simulink model "strelkowa_rep3_ODE"  (R2013a)
settings: Solver=ode4  StartTime=0.0  StopTime=3000.0  FixedStep=0.1  RelTol=1e-3
values from neighbouring files (symbols this model uses):
  c1 = P1(a)    [evaluation_ODE.m]    (also in init_Strelkowa_ODE.m = 1.6)
  c2 = 0.12    [evaluation_ODE.m]    (also in init_Strelkowa_ODE.m)
  c3 = 2.6    [evaluation_ODE.m]    (also in init_Strelkowa_ODE.m)
  c4 = 0.06    [evaluation_ODE.m]    (also in init_Strelkowa_ODE.m)
  mRNA_init = 10    [evaluation_ODE.m]    (also in init_Strelkowa_ODE.m)
settings Model: Creator=Jure Bordon  LastModifiedBy=Jure Bordon

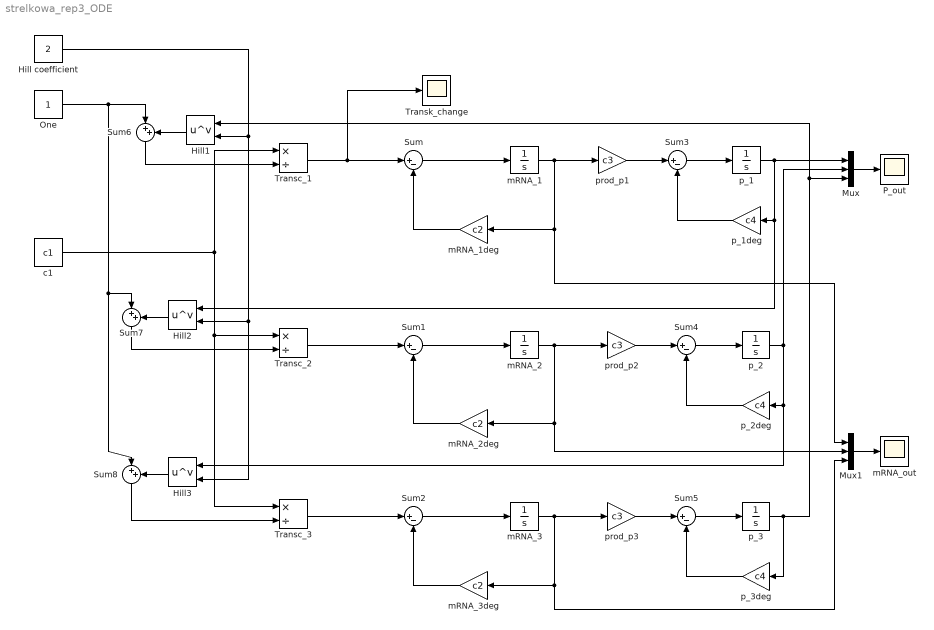
== system strelkowa_rep3_ODE ==
  Hill coefficient : Constant  Value=2
  Hill1 : Math  Operator=pow  SaturateOnIntegerOverflow=on
  Hill2 : Math  Operator=pow  SaturateOnIntegerOverflow=on
  Hill3 : Math  Operator=pow  SaturateOnIntegerOverflow=on
  Mux : Mux  Inputs=3
  Mux1 : Mux  Inputs=3
  One : Constant
  P_out : Scope
      settings: SaveName=P_out_ODE
  Sum{,1..5} (6 alike) : Sum  Inputs=|+-
  Sum6 : Sum  Inputs=|++
  Sum7 : Sum  Inputs=|++
  Sum8 : Sum  Inputs=|++
  Transc_1 : Product  Inputs=*/
  Transc_2 : Product  Inputs=*/
  Transc_3 : Product  Inputs=*/
  Transk_change : Scope
      settings: SaveName=P_out
  c1 : Constant  Value=c1
  mRNA_1 : Integrator  InitialCondition=mRNA_init + 0.5
  mRNA_1deg : Gain  Gain=c2
  mRNA_2 : Integrator  InitialCondition=mRNA_init
  mRNA_2deg : Gain  Gain=c2
  mRNA_3 : Integrator  InitialCondition=mRNA_init
  mRNA_3deg : Gain  Gain=c2
  mRNA_out : Scope
      settings: SaveName=mRNA_out_ODE
  p_1 : Integrator
  p_1deg : Gain  Gain=c4
  p_2 : Integrator
  p_2deg : Gain  Gain=c4
  p_3 : Integrator
  p_3deg : Gain  Gain=c4
  prod_p1 : Gain  Gain=c3
  prod_p2 : Gain  Gain=c3
  prod_p3 : Gain  Gain=c3
  wires:
  Sum/1 -> mRNA_1/1
  Sum1/1 -> mRNA_2/1
  Sum2/1 -> mRNA_3/1
  Sum3/1 -> p_1/1
  p_1/1 -> Mux/1, Hill2/1, p_1deg/1
  p_1deg/1 -> Sum3/2
  Sum4/1 -> p_2/1
  p_2/1 -> p_2deg/1, Hill3/1, Mux/2
  p_2deg/1 -> Sum4/2
  Sum5/1 -> p_3/1
  p_3/1 -> p_3deg/1, Hill1/1, Mux/3
  p_3deg/1 -> Sum5/2
  Sum6/1 -> Transc_1/2
  Sum8/1 -> Transc_3/2
  One/1 -> Sum7/1, Sum8/1, Sum6/1
  Transc_3/1 -> Sum2/1
  Transc_2/1 -> Sum1/1
  Transc_1/1 -> Transk_change/1, Sum/1
  Sum7/1 -> Transc_2/2
  c1/1 -> Transc_1/1, Transc_3/1, Transc_2/1
  Mux/1 -> P_out/1
  mRNA_1/1 -> prod_p1/1, Mux1/1, mRNA_1deg/1
  mRNA_2/1 -> prod_p2/1, Mux1/2, mRNA_2deg/1
  mRNA_3/1 -> mRNA_3deg/1, Mux1/3, prod_p3/1
  Mux1/1 -> mRNA_out/1
  mRNA_1deg/1 -> Sum/2
  mRNA_2deg/1 -> Sum1/2
  mRNA_3deg/1 -> Sum2/2
  prod_p1/1 -> Sum3/1
  prod_p3/1 -> Sum5/1
  prod_p2/1 -> Sum4/1
  Hill1/1 -> Sum6/2
  Hill2/1 -> Sum7/2
  Hill3/1 -> Sum8/2
  Hill coefficient/1 -> Hill3/2, Hill2/2, Hill1/2
